simulink model "Integrated_structure_for_speed_control"  (R2016b)
settings: Solver=FixedStepAuto  StartTime=0.0  StopTime=5  FixedStep=0.00001  RelTol=1e-3
settings Model: Creator=emilio  LastModifiedBy=danielesmn

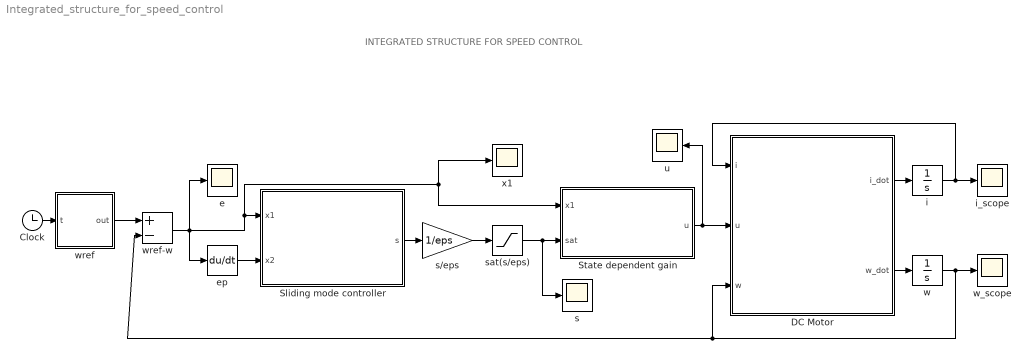
== system Integrated_structure_for_speed_control ==
  note: INTEGRATED STRUCTURE FOR SPEED CONTROL
  Clock : Clock
  DC Motor : MATLAB Function  TreatAsAtomicUnit=on
  Sliding mode controller : MATLAB Function  TreatAsAtomicUnit=on
  State dependent gain : MATLAB Function  TreatAsAtomicUnit=on
  e : Scope
  ep : Derivative
  i : Integrator
  i_scope : Scope
  s : Scope
  s/eps : Gain  Gain=1/eps
  sat(s/eps) : Saturate  UpperLimit=1  LowerLimit=-1  ZeroCross=off
  u : Scope
  w : Integrator
  w_scope : Scope
  wref : MATLAB Function  TreatAsAtomicUnit=on
  wref-w : Sum  Inputs=+-
  x1 : Scope
  wires:
  wref-w/1 -> Sliding mode controller/1(x1), x1/1, State dependent gain/1(x1), e/1, ep/1
  wref/1(out) -> wref-w/1
  ep/1 -> Sliding mode controller/2(x2)
  Clock/1 -> wref/1(t)
  DC Motor/1(i_dot) -> i/1
  DC Motor/2(w_dot) -> w/1
  w/1 -> DC Motor/3(w), wref-w/2, w_scope/1
  i/1 -> DC Motor/1(i), i_scope/1
  s/eps/1 -> sat(s/eps)/1
  Sliding mode controller/1(s) -> s/eps/1
  State dependent gain/1(u) -> DC Motor/2(u), u/1
  sat(s/eps)/1 -> s/1, State dependent gain/2(sat)

== matlab function Integrated_structure_for_speed_control/State dependent gain ==
  data: x1 input; u output; sat input
function u = SDG(x1, sat)

u0 = 1;
delta = 10;

u = (u0 + delta*abs(x1))*sat;

== matlab function Integrated_structure_for_speed_control/Sliding mode controller ==
  data: x1 input; x2 input; s output
function s = SMC(x1, x2)

c = 30;

s = c*x1 + x2; %Sliding surface

== matlab function Integrated_structure_for_speed_control/wref ==
  data: t input; out output
function out = input(t)

if t > 2 && t < 3.5
    out = 1;
else
    out = -1;
end

== matlab function Integrated_structure_for_speed_control/DC Motor ==
  data: i input; i_dot output; u input; w input; w_dot output
function [i_dot, w_dot] = Dc_Motor(i, u, w) % i: armature current w: shaft speed

%% Model of the DC Motor

L = 0.001;        %Armature inductance (H)
R = 0.5;          %Armature resistance (Ohm)
kt = 0.008;       %Torque constant (Nm/A)
J = 0.001;        %Inertia of the motor rotor (Kg*m^2)
B = 0.01;         %Coefficient of viscous friction (Nm*s/rad)
lambda0 = 0.001;  %Back electromotive force (EMF) constant (V*s/rad)

tauL = B*w;        %Load torque

i_dot = u/L - R/L*i - lambda0/L*w;      %Electrical part model
w_dot = (kt*i - tauL)/J;              %Mechanical part model
